simulink model "MPG_MG_freq"  (R2021b)
settings: Solver=VariableStepAuto  StartTime=0.0  StopTime=7  RelTol=1e-3
model workspace (MAT data in the model file):
  Ts : Simulink.Parameter (value not decoded)
  secondary_on : Simulink.Parameter (value not decoded)
values from neighbouring files (symbols this model uses):
  A = zeros(4,4)    [MPC_MG_script_raw_dmpc.m]    (also in MPG_MG_July.m = [0 1 1 1; 1 0 0 0; 1 0 0 0; 1 0 0 0]; MPG_MG_freq_script.m = ones(4) - eye(4); Script.m = [0 1 1 1 ; 1 0 1 1 ; 1 1 0 1 ; 1 1 1 0])
  C_f = 50e-6    (= 5e-05)    [Four_DG_MG_PrimaryOnlyScript.m]    (also in MPC_MG_script.m; MPC_MG_script_raw_dmpc.m; MPC_MG_secondary_script.m; MPG_MG_July.m)
  f_c = 5000    [Four_DG_MG_PrimaryOnlyScript.m]    (also in MPC_MG_script.m = 40000; MPC_MG_script_raw_dmpc.m = 40000; MPC_MG_secondary_script.m = 40000; MPG_MG_July.m = 50000)
  kL = 1e-5    (= 1e-05)    [Four_DG_MG_PrimaryOnlyScript.m]    (also in MPC_MG_script.m = 1e-08; MPC_MG_script_raw_dmpc.m = 1e-08; MPC_MG_secondary_script.m = 1e-07; MPG_MG_July.m = 1e-07)
  L_f = 1.35e-3    (= 0.00135)    [Four_DG_MG_PrimaryOnlyScript.m]    (also in MPC_MG_script.m; MPC_MG_script_raw_dmpc.m; MPC_MG_secondary_script.m; MPG_MG_July.m)
  L_in1 = 0.35e-3    (= 0.00035)    [Four_DG_MG_PrimaryOnlyScript.m]    (also in MPC_MG_script.m; MPC_MG_script_raw_dmpc.m; MPC_MG_secondary_script.m; MPG_MG_July.m)
  L_in2 = 0.35e-3    (= 0.00035)    [Four_DG_MG_PrimaryOnlyScript.m]    (also in MPC_MG_script.m; MPC_MG_script_raw_dmpc.m; MPC_MG_secondary_script.m; MPG_MG_July.m)
  L_in4 = 0.35e-3    (= 0.00035)    [Four_DG_MG_PrimaryOnlyScript.m]    (also in MPC_MG_script.m; MPC_MG_script_raw_dmpc.m; MPC_MG_secondary_script.m; MPG_MG_July.m)
  lambda1 = [30000 50000 90000 50000]'    [MPC_MG_script_raw_dmpc.m]    (also in MPG_MG_July.m = [4 4 4 4]'; MPG_MG_freq_script.m = [3 3 3 3]'; Script.m = [1 1 1 1]')
  lambda2 = [5 6 7 6]'    [MPC_MG_script_raw_dmpc.m]    (also in MPG_MG_July.m = [0.5e-2 0.5e-2 0.5e-2 0.5e-2]'; MPG_MG_freq_script.m = [1.1 1.9 1.5 1.2]'; Script.m = [0.8e-2 0.8e-2 0.8e-2 0.8e-2]')
  lambda3 = [80000 80000 900000 80000]'    [MPC_MG_script_raw_dmpc.m]    (also in MPG_MG_July.m = [1e-3 1e-3 1e-3 1e-3]'; MPG_MG_freq_script.m = [9e-4 1.2e-2 3e-3 3e-3]'; Script.m = [1.5e-3 1.5e-3 1.5e-3 1.5e-3]')
  LD_ref1 = 800e-6    (= 0.0008)    [Four_DG_MG_PrimaryOnlyScript.m]    (also in MPC_MG_script.m = 0.0003; MPC_MG_script_raw_dmpc.m = 0.0003; MPC_MG_secondary_script.m = 0.0001; MPG_MG_July.m = 0.0004)
  lo_co = 0.2    [Four_DG_MG_PrimaryOnlyScript.m]    (also in MPC_MG_script.m = 0.05; MPC_MG_script_raw_dmpc.m; MPC_MG_secondary_script.m = 0.08; MPG_MG_July.m = 0.15)
  m_p1 = 9.4e-5/droopDivide    (= 9.4e-05)    [Four_DG_MG_PrimaryOnlyScript.m]    (also in MPC_MG_script.m; MPC_MG_script_raw_dmpc.m; MPC_MG_secondary_script.m; MPG_MG_July.m)
  m_p2 = 9.4e-5/droopDivide    (= 9.4e-05)    [Four_DG_MG_PrimaryOnlyScript.m]    (also in MPC_MG_script.m; MPC_MG_script_raw_dmpc.m; MPC_MG_secondary_script.m; MPG_MG_July.m)
  m_p3 = 12.5e-5/droopDivide    (= 0.000125)    [Four_DG_MG_PrimaryOnlyScript.m]    (also in MPC_MG_script.m; MPC_MG_script_raw_dmpc.m; MPC_MG_secondary_script.m; MPG_MG_July.m)
  m_p4 = 12.5e-5/droopDivide    (= 0.000125)    [Four_DG_MG_PrimaryOnlyScript.m]    (also in MPC_MG_script.m; MPC_MG_script_raw_dmpc.m; MPC_MG_secondary_script.m; MPG_MG_July.m)
  N = 3    [MPG_MG_July.m]    (also in MPG_MG_freq_script.m; Script.m = 5)
  n_q1 = 1.3e-3/droopDivide2    (= 0.00013)    [Four_DG_MG_PrimaryOnlyScript.m]    (also in MPC_MG_script.m; MPC_MG_script_raw_dmpc.m; MPC_MG_secondary_script.m; MPG_MG_July.m)
  n_q2 = 1.3e-3/droopDivide2    (= 0.00013)    [Four_DG_MG_PrimaryOnlyScript.m]    (also in MPC_MG_script.m; MPC_MG_script_raw_dmpc.m; MPC_MG_secondary_script.m; MPG_MG_July.m)
  n_q4 = 1.5e-3/droopDivide2    (= 0.00015)    [Four_DG_MG_PrimaryOnlyScript.m]    (also in MPC_MG_script.m; MPC_MG_script_raw_dmpc.m; MPC_MG_secondary_script.m; MPG_MG_July.m)
  Pmax = [45e3 45e3 37e3 37e3]'    [MPG_MG_July.m]    (also in MPG_MG_freq_script.m = [4e3 3.5e3 3.5e3 4e3]'; Script.m)
  R_f = 0.1    [Four_DG_MG_PrimaryOnlyScript.m]    (also in MPC_MG_script.m; MPC_MG_script_raw_dmpc.m; MPC_MG_secondary_script.m; MPG_MG_July.m)
  R_in1 = 0.03    [Four_DG_MG_PrimaryOnlyScript.m]    (also in MPC_MG_script.m; MPC_MG_script_raw_dmpc.m; MPC_MG_secondary_script.m; MPG_MG_July.m)
  R_in2 = 0.03    [Four_DG_MG_PrimaryOnlyScript.m]    (also in MPC_MG_script.m; MPC_MG_script_raw_dmpc.m; MPC_MG_secondary_script.m; MPG_MG_July.m)
  R_in4 = 0.03    [Four_DG_MG_PrimaryOnlyScript.m]    (also in MPC_MG_script.m; MPC_MG_script_raw_dmpc.m; MPC_MG_secondary_script.m; MPG_MG_July.m)
  time_thresh = 0.6    [Four_DG_MG_PrimaryOnlyScript.m]    (also in MPC_MG_script_raw_dmpc.m = 1.5; MPC_MG_secondary_script.m = 2; MPG_MG_July.m = 0.5; MPG_MG_freq_script.m = 0.5)
  Ts = 10e-6    (= 1e-05)    [Four_DG_MG_PrimaryOnlyScript.m]    (also in MPC_MG_script.m; MPC_MG_script_raw_dmpc.m; MPC_MG_secondary_script.m; MPG_MG_July.m)
  Tsamp = 0.1    [MPG_MG_July.m]    (also in MPG_MG_freq_script.m; Script.m)
  V_nom = 220*sqrt(2)    [Four_DG_MG_PrimaryOnlyScript.m]    (also in MPC_MG_script.m; MPC_MG_script_raw_dmpc.m; MPC_MG_secondary_script.m; MPG_MG_July.m)
  Vdc = 600    [Four_DG_MG_PrimaryOnlyScript.m]    (also in MPC_MG_script.m; MPC_MG_script_raw_dmpc.m; MPC_MG_secondary_script.m; MPG_MG_July.m)
  w_c_high = 2*pi*50    (= 314.159265359)    [Four_DG_MG_PrimaryOnlyScript.m]    (also in MPC_MG_script.m; MPC_MG_script_raw_dmpc.m; MPC_MG_secondary_script.m; MPG_MG_July.m)
  w_nom = 2*pi*50    (= 314.159265359)    [Four_DG_MG_PrimaryOnlyScript.m]    (also in MPC_MG_script.m; MPC_MG_script_raw_dmpc.m; MPC_MG_secondary_script.m; MPG_MG_July.m)
undefined symbols (not defined in the file or in its folder): i
libraries: spsThreePhaseSeriesRLCBranchLib x18, spsabctodq0Lib x16, spsThreePhaseVIMeasurementLib x15, eeGeneralControl x14, dspswit3 x5, spsDCVoltageSourceLib x5, spsSeriesRLCBranchLib x5, spsTwoLevelConverterLib x5, slpidlib x4, spsThreePhaseSeriesRLCLoadLib x2, spsThreePhaseBreakerLib x2, spsPLL3phLib x2
(part 4 of 4)

== matlab function MPG_MG_freq/Voltage Source Inverter 2/Model Predictive Control  ==
  settings: updateMethod=DISCRETE  sampleTime=Ts
  data: S_opt output; Sopt output size=[1 6]; Vc input; i_filter input; vref input; Vi_opt output; Vdc parameter double size=1; modT parameter size=1; Cfilter parameter size=1; Lfilter parameter size=1
function [S_opt, Sopt, Vi_opt] = MPC(Vc, i_filter,vref,Vdc,modT,Cfilter,Lfilter)

    % In order to call "cont2dis" function
    coder.extrinsic('cont2dis');
    persistent Aq Bq Bdq Vck ifk  Vc_old if_old x_opt g f_window f_window2

    % Initialize variables and get the parameters of the Discrete model based on Ts
    if isempty(x_opt), x_opt = ones(1, 2); end
    if isempty(Vc_old), Vc_old = 0 + 1j*0; end
    if isempty(if_old), if_old = 0 + 1j*0; end
    if isempty(Vck), Vck = ones(1, 4) * (0 + 1j*0); end
    if isempty(ifk), ifk = ones(1, 4) * (0 + 1j*0); end
    if isempty(f_window), f_window = zeros(1,51); end
    if isempty(f_window2), f_window2 = zeros(1,51); end

    if isempty(Aq) && isempty(Bq) && isempty(Bdq)
        Aq = zeros(2);     Bq = zeros(2,1);     Bdq = zeros(2,1);
        % Call "cont2dis" function
        [Aq, Bq, Bdq] = cont2dis(modT,Lfilter,Cfilter); 
    end
    
    % Intialize the cost function
    g_opt = inf;
    
    % To generate the switching states matrix
    states = [1 0 0;
              0 0 0  
              1 1 0
              0 1 0
              0 1 1
              0 0 1
              1 0 1
              1 1 1];
    a = exp(1j*(2*pi/3));
    % Read current measurements at sampling instant k
    ifk(1) = i_filter;
    Vck(1) = Vc;
    % Equation of io(k-1) = if(k-1)-(c/Ts)(vc(k)-vc(k-1)).
    io = ones(1, 3) * (0 + 1j*0);
    io(1) = if_old - (Cfilter/modT)*(Vck(1) - Vc_old); 
    
    % Store the measured current for the next iteration
    if_old = i_filter;
    Vc_old = Vc;
    % FOR loop to find the best switch in the next instant and its corresponding V(i)
    k = ones(1,3);
    s = zeros(3,3);
    sw = zeros(1,3)* (0 + 1j*0);
    Vi = zeros(1,3)* (0 + 1j*0);
    for a1 = 1:8
        k(1) = a1;
        %constraint check
        if (abs(states(k(1),:)-states(x_opt(1),:)) > 1)
            continue
        end
        %state calculation
        s(1,:) = states(k(1),:);
        sw(1) = (2/3)*(s(1,1)+a*s(1,2)+a^2*s(1,3));
        Vi(1) = Vdc*sw(1);

        % Output Voltage Prediction at instant k+1
        ifk(2) = Aq(1,1)*ifk(1) + Aq(1,2)*Vck(1) + Bq(1)*Vi(1) + Bdq(1)*io(1); 
        Vck(2) = Aq(2,1)*ifk(1) + Aq(2,2)*Vck(1) + Bq(2)*Vi(1) + Bdq(2)*io(1); 
        
        for a2 = 1:8
            k(2) = a2;
            %constraint check
            if (abs(states(k(2),:)-states(k(1),:)) > 1)
                continue
            end
            io(2) = io(1) - (Cfilter/modT)*(Vck(2) - Vck(1));
            %state calculation
            s(2,:) = states(k(2),:);
            sw(2) = (2/3)*(s(2,1)+a*s(2,2)+a^2*s(2,3));
            Vi(2) = Vdc*sw(2);
    
            % Output Voltage Prediction at instant k+1
            ifk(3) = Aq(1,1)*ifk(2) + Aq(1,2)*Vck(2) + Bq(1)*Vi(2) + Bdq(1)*io(2); 
            Vck(3) = Aq(2,1)*ifk(2) + Aq(2,2)*Vck(2) + Bq(2)*Vi(2) + Bdq(2)*io(2); 

            g1 = (real(ifk(3))-real(io(3))+Cfilter*2*pi*50*imag(vref))^2 + (imag(ifk(3))-imag(io(3))+Cfilter*2*pi*50*real(vref))^2;
            g = (real(vref)-real(Vck(3)))^2+(imag(vref)-imag(Vck(3)))^2 + 0.1*g1 + 0.1*sum(states(a2)-states(a1),'all')^2;
            if (g<g_opt)
                x_opt = [k(1) k(2)];
                g_opt = g;
            end
           
        end 
    end

     
    
    % Output switching states and its voltage vector. 
    Vi_opt = x_opt(1); 
    S_opt = states(x_opt(1),:);
    d_opt = not(S_opt);
    Sopt = [S_opt,d_opt];     

end

== matlab function MPG_MG_freq/Voltage Source Inverter 1/Model Predictive Control  ==
  settings: updateMethod=DISCRETE  sampleTime=Ts
  data: Sopt output size=[1 6]; Vc input; i_filter input; vref input; Vdc parameter double size=1; modT parameter size=1; Cfilter parameter size=1; Lfilter parameter size=1
function Sopt  = MPC(Vc, i_filter,vref,Vdc,modT,Cfilter,Lfilter)

    % In order to call "cont2dis" function
    coder.extrinsic('cont2dis');
    persistent Aq Bq Bdq Vck ifk  Vc_old if_old x_opt g f_window f_window2

    % Initialize variables and get the parameters of the Discrete model based on Ts
    if isempty(x_opt), x_opt = ones(1, 2); end
    if isempty(Vc_old), Vc_old = 0 + 1j*0; end
    if isempty(if_old), if_old = 0 + 1j*0; end
    if isempty(Vck), Vck = ones(1, 4) * (0 + 1j*0); end
    if isempty(ifk), ifk = ones(1, 4) * (0 + 1j*0); end
    if isempty(f_window), f_window = zeros(1,51); end
    if isempty(f_window2), f_window2 = zeros(1,51); end

    if isempty(Aq) && isempty(Bq) && isempty(Bdq)
        Aq = zeros(2);     Bq = zeros(2,1);     Bdq = zeros(2,1);
        % Call "cont2dis" function
        [Aq, Bq, Bdq] = cont2dis(modT,Lfilter,Cfilter); 
    end
    
    % Intialize the cost function
    g_opt = inf;
    
    % To generate the switching states matrix
    states = [1 0 0;
              0 0 0  
              1 1 0
              0 1 0
              0 1 1
              0 0 1
              1 0 1
              1 1 1];
    a = exp(1j*(2*pi/3));
    % Read current measurements at sampling instant k
    ifk(1) = i_filter;
    Vck(1) = Vc;
    % Equation of io(k-1) = if(k-1)-(c/Ts)(vc(k)-vc(k-1)).
    io = ones(1, 3) * (0 + 1j*0);
    io(1) = if_old - (Cfilter/modT)*(Vck(1) - Vc_old); 
    
    % Store the measured current for the next iteration
    if_old = i_filter;
    Vc_old = Vc;
    % FOR loop to find the best switch in the next instant and its corresponding V(i)
    k = ones(1,3);
    s = zeros(3,3);
    sw = zeros(1,3)* (0 + 1j*0);
    Vi = zeros(1,3)* (0 + 1j*0);
    for a1 = 1:8
        k(1) = a1;
        %constraint check
        if (abs(states(k(1),:)-states(x_opt(1),:)) > 1)
            continue
        end
        %state calculation
        s(1,:) = states(k(1),:);
        sw(1) = (2/3)*(s(1,1)+a*s(1,2)+a^2*s(1,3));
        Vi(1) = Vdc*sw(1);

        % Output Voltage Prediction at instant k+1
        ifk(2) = Aq(1,1)*ifk(1) + Aq(1,2)*Vck(1) + Bq(1)*Vi(1) + Bdq(1)*io(1); 
        Vck(2) = Aq(2,1)*ifk(1) + Aq(2,2)*Vck(1) + Bq(2)*Vi(1) + Bdq(2)*io(1); 
        
        for a2 = 1:8
            k(2) = a2;
            %constraint check
            if (abs(states(k(2),:)-states(k(1),:)) > 1)
                continue
            end
            io(2) = io(1) - (Cfilter/modT)*(Vck(2) - Vck(1));
            %state calculation
            s(2,:) = states(k(2),:);
            sw(2) = (2/3)*(s(2,1)+a*s(2,2)+a^2*s(2,3));
            Vi(2) = Vdc*sw(2);
    
            % Output Voltage Prediction at instant k+1
            ifk(3) = Aq(1,1)*ifk(2) + Aq(1,2)*Vck(2) + Bq(1)*Vi(2) + Bdq(1)*io(2); 
            Vck(3) = Aq(2,1)*ifk(2) + Aq(2,2)*Vck(2) + Bq(2)*Vi(2) + Bdq(2)*io(2); 

            g1 = (real(ifk(3))-real(io(3))+Cfilter*2*pi*50*imag(vref))^2 + (imag(ifk(3))-imag(io(3))+Cfilter*2*pi*50*real(vref))^2;
            g = (real(vref)-real(Vck(3)))^2+(imag(vref)-imag(Vck(3)))^2 + 0.1*g1;
            if (g<g_opt)
                x_opt = [k(1) k(2)];
                g_opt = g;
            end
           
        end 
    end

     
    
    % Output switching states and its voltage vector. 
    Vi_opt = x_opt(1); 
    S_opt = states(x_opt(1),:);
    d_opt = not(S_opt);
    Sopt = [S_opt,d_opt];     

end

== matlab function MPG_MG_freq/Voltage Source Inverter 3/Model Predictive Control  ==
  settings: updateMethod=DISCRETE  sampleTime=Ts
  data: S_opt output; Sopt output size=[1 6]; Vc input; i_filter input; vref input; Vi_opt output; Vdc parameter double size=1; modT parameter size=1; Cfilter parameter size=1; Lfilter parameter size=1
function [S_opt, Sopt, Vi_opt] = MPC(Vc, i_filter,vref,Vdc,modT,Cfilter,Lfilter)

    % In order to call "cont2dis" function
    coder.extrinsic('cont2dis');
    persistent Aq Bq Bdq Vck ifk  Vc_old if_old x_opt g f_window f_window2

    % Initialize variables and get the parameters of the Discrete model based on Ts
    if isempty(x_opt), x_opt = ones(1, 2); end
    if isempty(Vc_old), Vc_old = 0 + 1j*0; end
    if isempty(if_old), if_old = 0 + 1j*0; end
    if isempty(Vck), Vck = ones(1, 4) * (0 + 1j*0); end
    if isempty(ifk), ifk = ones(1, 4) * (0 + 1j*0); end
    if isempty(f_window), f_window = zeros(1,51); end
    if isempty(f_window2), f_window2 = zeros(1,51); end

    if isempty(Aq) && isempty(Bq) && isempty(Bdq)
        Aq = zeros(2);     Bq = zeros(2,1);     Bdq = zeros(2,1);
        % Call "cont2dis" function
        [Aq, Bq, Bdq] = cont2dis(modT,Lfilter,Cfilter); 
    end
    
    % Intialize the cost function
    g_opt = inf;
    
    % To generate the switching states matrix
    states = [1 0 0;
              0 0 0  
              1 1 0
              0 1 0
              0 1 1
              0 0 1
              1 0 1
              1 1 1];
    a = exp(1j*(2*pi/3));
    % Read current measurements at sampling instant k
    ifk(1) = i_filter;
    Vck(1) = Vc;
    % Equation of io(k-1) = if(k-1)-(c/Ts)(vc(k)-vc(k-1)).
    io = ones(1, 3) * (0 + 1j*0);
    io(1) = if_old - (Cfilter/modT)*(Vck(1) - Vc_old); 
    
    % Store the measured current for the next iteration
    if_old = i_filter;
    Vc_old = Vc;
    % FOR loop to find the best switch in the next instant and its corresponding V(i)
    k = ones(1,3);
    s = zeros(3,3);
    sw = zeros(1,3)* (0 + 1j*0);
    Vi = zeros(1,3)* (0 + 1j*0);
    for a1 = 1:8
        k(1) = a1;
        %constraint check
        if (abs(states(k(1),:)-states(x_opt(1),:)) > 1)
            continue
        end
        %state calculation
        s(1,:) = states(k(1),:);
        sw(1) = (2/3)*(s(1,1)+a*s(1,2)+a^2*s(1,3));
        Vi(1) = Vdc*sw(1);

        % Output Voltage Prediction at instant k+1
        ifk(2) = Aq(1,1)*ifk(1) + Aq(1,2)*Vck(1) + Bq(1)*Vi(1) + Bdq(1)*io(1); 
        Vck(2) = Aq(2,1)*ifk(1) + Aq(2,2)*Vck(1) + Bq(2)*Vi(1) + Bdq(2)*io(1); 
        
        for a2 = 1:8
            k(2) = a2;
            %constraint check
            if (abs(states(k(2),:)-states(k(1),:)) > 1)
                continue
            end
            io(2) = io(1) - (Cfilter/modT)*(Vck(2) - Vck(1));
            %state calculation
            s(2,:) = states(k(2),:);
            sw(2) = (2/3)*(s(2,1)+a*s(2,2)+a^2*s(2,3));
            Vi(2) = Vdc*sw(2);
    
            % Output Voltage Prediction at instant k+1
            ifk(3) = Aq(1,1)*ifk(2) + Aq(1,2)*Vck(2) + Bq(1)*Vi(2) + Bdq(1)*io(2); 
            Vck(3) = Aq(2,1)*ifk(2) + Aq(2,2)*Vck(2) + Bq(2)*Vi(2) + Bdq(2)*io(2); 

            g1 = (real(ifk(3))-real(io(3))+Cfilter*2*pi*50*imag(vref))^2 + (imag(ifk(3))-imag(io(3))+Cfilter*2*pi*50*real(vref))^2;
            g = (real(vref)-real(Vck(3)))^2+(imag(vref)-imag(Vck(3)))^2 + 0.1*g1 + 0.1*sum(states(a2)-states(a1),'all')^2;
            if (g<g_opt)
                x_opt = [k(1) k(2)];
                g_opt = g;
            end
           
        end 
    end

     
    
    % Output switching states and its voltage vector. 
    Vi_opt = x_opt(1); 
    S_opt = states(x_opt(1),:);
    d_opt = not(S_opt);
    Sopt = [S_opt,d_opt];     

end

== matlab function MPG_MG_freq/MPC-based Secondary Controller/Subsystem1/Model Predictive Control 1 ==
  settings: updateMethod=DISCRETE  sampleTime=Ts
  data: flag output; X input; a input; x_out output; L_f input; Mpw input; Tsec input; omega input; omega_s input; V input; V_s input; theta input; P input; w_nom input; lambda1 input; lambda2 input; lambda3 input; Pmax input; aij input; N parameter
function [flag, x_out] = dmpc(X, a, L_f, Mpw, Tsec, omega, omega_s, V, V_s, theta, P, w_nom, lambda1, lambda2, lambda3, Pmax, aij, N)
    %step 5: update matrices
   
    Ai = zeros(2*N,5*N);

    Ai(1:N,(4*N+1):5*N) = -eye(N);
    Ai((1*N+1):2*N,(4*N+1):5*N) = eye(N);

    Bi = zeros((2*N),1);

    Bi((1+N):(2*N),1) = Pmax(a)*ones(N,1);

    tz = toeplitz([1 -1 zeros(1,N-2)], [1 zeros(1,N-1)]);

    Aeq = zeros(4*N,5*N);

    Aeq((N+1):2*N, (N+1):(2*N)) = -eye(N);
    Aeq((N+1):2*N, (2*N+1):3*N) = tz;
    Aeq((N+1):2*N, (4*N+1):5*N) =  -Mpw*tz;

    Aeq((2*N+1):(3*N), (2*N+1):(3*N)) = -Tsec*eye(N); 
    Aeq((2*N+1):(3*N), (3*N+1):4*N) = tz;

    Aeq((3*N+1):(4*N), (3*N+1):(4*N)) = -V(a)*V_s(a)*cos(theta(a))/(L_f*w_nom)*eye(N);
    Aeq((3*N+1):(4*N), (4*N+1):5*N) = eye(N);

    I9 = eye(N);
    I9(N,N) = 0;

    Aeq(1:N, 1:N) = eye(N);
    Aeq(1:N, (2*N+1):(3*N)) = -1/(1+sum(aij(a,:)))*I9;
   
    Beq = zeros(4*N,1);

    Beq(1:N,1) = (aij(a,:)*X(:,(2*N+1):3*N)./(1+sum(aij(a,:))))';

    Beq(N+1,1) = omega(a)-Mpw*P(a);

    Beq((2*N+1),1) = theta(a)-Tsec*omega_s(a);
    Beq((2*N+2):(3*N),1) = -Tsec*omega_s(a)*ones((N-1),1);

    Beq((3*N+1):(4*N),1) = (P(a)-theta(a)*V(a)*V_s(a)*cos(theta(a))/(L_f*w_nom))*ones(N,1);
    
    H = zeros(5*N);
    H(1:N,1:N) = 2*lambda1(a)*eye(N);
    H((N+1):(2*N),(N+1):(2*N)) = 2*lambda2(a)*eye(N);
    H((4*N+1):5*N,(4*N+1):5*N) = 2*lambda3(a)*sum(aij(a,:))/(Pmax(a)^2)*eye(N);

    S_pred = ones(4,N);
    for k = 1:N
        S_pred(:,k) = Pmax; 
    end

    F = zeros(5*N,1);
    F(1:N,1) = -2*lambda1(a)*w_nom*ones(N,1);

    F((4*N+1):5*N,1) = -2*lambda3(a)*(aij(a,:)*(X(:,(4*N+1):5*N)./(S_pred))/Pmax(a))';
    %P_pred 4x10 matrix
    options = optimoptions('quadprog', 'Algorithm','active-set');
    %required initial point x0
    %   OPTIMIZE
    x0 = zeros(5*N,1);
    x0(1,1) = w_nom;
    x0((N+1),1) = 0;
    x0((2*N+1),1) = w_nom;
    x0((3*N+1),1) = 0.963;
    x0((4*N+1),1) = 0;

    [x,~,exitflag] = quadprog(H, F, Ai, Bi, Aeq, Beq, [], [], x0, options);
    x_out = x;

    if exitflag < 1
       x((N+1),1) = 0;
    else
        x_out = x;
    end
    flag = exitflag;
end

== matlab function MPG_MG_freq/MPC-based Secondary Controller/Subsystem6/Model Predictive Control 1 ==
  settings: updateMethod=DISCRETE  sampleTime=Ts
  data: flag output; X input; a input; x_out output; L_f input; Mpw input; Tsec input; omega input; omega_s input; V input; V_s input; theta input; P input; w_nom input; lambda1 input; lambda2 input; lambda3 input; Pmax input; aij input; N parameter
function [flag, x_out] = dmpc(X, a, L_f, Mpw, Tsec, omega, omega_s, V, V_s, theta, P, w_nom, lambda1, lambda2, lambda3, Pmax, aij, N)
    %step 5: update matrices
   
    Ai = zeros(2*N,5*N);

    Ai(1:N,(4*N+1):5*N) = -eye(N);
    Ai((1*N+1):2*N,(4*N+1):5*N) = eye(N);

    Bi = zeros((2*N),1);

    Bi((1+N):(2*N),1) = Pmax(a)*ones(N,1);

    tz = toeplitz([1 -1 zeros(1,N-2)], [1 zeros(1,N-1)]);

    Aeq = zeros(4*N,5*N);

    Aeq((N+1):2*N, (N+1):(2*N)) = -eye(N);
    Aeq((N+1):2*N, (2*N+1):3*N) = tz;
    Aeq((N+1):2*N, (4*N+1):5*N) =  -Mpw*tz;

    Aeq((2*N+1):(3*N), (2*N+1):(3*N)) = -Tsec*eye(N); 
    Aeq((2*N+1):(3*N), (3*N+1):4*N) = tz;

    Aeq((3*N+1):(4*N), (3*N+1):(4*N)) = -V(a)*V_s(a)*cos(theta(a))/(L_f*w_nom)*eye(N);
    Aeq((3*N+1):(4*N), (4*N+1):5*N) = eye(N);

    I9 = eye(N);
    I9(N,N) = 0;

    Aeq(1:N, 1:N) = eye(N);
    Aeq(1:N, (2*N+1):(3*N)) = -1/(1+sum(aij(a,:)))*I9;
   
    Beq = zeros(4*N,1);

    Beq(1:N,1) = (aij(a,:)*X(:,(2*N+1):3*N)./(1+sum(aij(a,:))))';

    Beq(N+1,1) = omega(a)-Mpw*P(a);

    Beq((2*N+1),1) = theta(a)-Tsec*omega_s(a);
    Beq((2*N+2):(3*N),1) = -Tsec*omega_s(a)*ones((N-1),1);

    Beq((3*N+1):(4*N),1) = (P(a)-theta(a)*V(a)*V_s(a)*cos(theta(a))/(L_f*w_nom))*ones(N,1);
    
    H = zeros(5*N);
    H(1:N,1:N) = 2*lambda1(a)*eye(N);
    H((N+1):(2*N),(N+1):(2*N)) = 2*lambda2(a)*eye(N);
    H((4*N+1):5*N,(4*N+1):5*N) = 2*lambda3(a)*sum(aij(a,:))/(Pmax(a)^2)*eye(N);

    S_pred = ones(4,N);
    for k = 1:N
        S_pred(:,k) = Pmax; 
    end

    F = zeros(5*N,1);
    F(1:N,1) = -2*lambda1(a)*w_nom*ones(N,1);

    F((4*N+1):5*N,1) = -2*lambda3(a)*(aij(a,:)*(X(:,(4*N+1):5*N)./(S_pred))/Pmax(a))';
    %P_pred 4x10 matrix
    options = optimoptions('quadprog', 'Algorithm','active-set');
    %required initial point x0
    %   OPTIMIZE
    x0 = zeros(5*N,1);
    x0(1,1) = w_nom;
    x0((N+1),1) = 0;
    x0((2*N+1),1) = w_nom;
    x0((3*N+1),1) = 0.963;
    x0((4*N+1),1) = 0;

    [x,~,exitflag] = quadprog(H, F, Ai, Bi, Aeq, Beq, [], [], x0, options);
    x_out = x;

    if exitflag < 1
       x((N+1),1) = 0;
    else
        x_out = x;
    end
    flag = exitflag;
end

== matlab function MPG_MG_freq/Voltage Source Inverter 4/Model Predictive Control  ==
  settings: updateMethod=DISCRETE  sampleTime=Ts
  data: S_opt output; Sopt output size=[1 6]; Vc input; i_filter input; vref input; Vi_opt output; Vdc parameter double size=1; modT parameter size=1; Cfilter parameter size=1; Lfilter parameter size=1
function [S_opt, Sopt, Vi_opt] = MPC(Vc, i_filter,vref,Vdc,modT,Cfilter,Lfilter)

    % In order to call "cont2dis" function
    coder.extrinsic('cont2dis');
    persistent Aq Bq Bdq Vck ifk  Vc_old if_old x_opt g f_window f_window2

    % Initialize variables and get the parameters of the Discrete model based on Ts
    if isempty(x_opt), x_opt = ones(1, 2); end
    if isempty(Vc_old), Vc_old = 0 + 1j*0; end
    if isempty(if_old), if_old = 0 + 1j*0; end
    if isempty(Vck), Vck = ones(1, 4) * (0 + 1j*0); end
    if isempty(ifk), ifk = ones(1, 4) * (0 + 1j*0); end
    if isempty(f_window), f_window = zeros(1,51); end
    if isempty(f_window2), f_window2 = zeros(1,51); end

    if isempty(Aq) && isempty(Bq) && isempty(Bdq)
        Aq = zeros(2);     Bq = zeros(2,1);     Bdq = zeros(2,1);
        % Call "cont2dis" function
        [Aq, Bq, Bdq] = cont2dis(modT,Lfilter,Cfilter); 
    end
    
    % Intialize the cost function
    g_opt = inf;
    
    % To generate the switching states matrix
    states = [1 0 0;
              0 0 0  
              1 1 0
              0 1 0
              0 1 1
              0 0 1
              1 0 1
              1 1 1];
    a = exp(1j*(2*pi/3));
    % Read current measurements at sampling instant k
    ifk(1) = i_filter;
    Vck(1) = Vc;
    % Equation of io(k-1) = if(k-1)-(c/Ts)(vc(k)-vc(k-1)).
    io = ones(1, 3) * (0 + 1j*0);
    io(1) = if_old - (Cfilter/modT)*(Vck(1) - Vc_old); 
    
    % Store the measured current for the next iteration
    if_old = i_filter;
    Vc_old = Vc;
    % FOR loop to find the best switch in the next instant and its corresponding V(i)
    k = ones(1,3);
    s = zeros(3,3);
    sw = zeros(1,3)* (0 + 1j*0);
    Vi = zeros(1,3)* (0 + 1j*0);
    for a1 = 1:8
        k(1) = a1;
        %constraint check
        if (abs(states(k(1),:)-states(x_opt(1),:)) > 1)
            continue
        end
        %state calculation
        s(1,:) = states(k(1),:);
        sw(1) = (2/3)*(s(1,1)+a*s(1,2)+a^2*s(1,3));
        Vi(1) = Vdc*sw(1);

        % Output Voltage Prediction at instant k+1
        ifk(2) = Aq(1,1)*ifk(1) + Aq(1,2)*Vck(1) + Bq(1)*Vi(1) + Bdq(1)*io(1); 
        Vck(2) = Aq(2,1)*ifk(1) + Aq(2,2)*Vck(1) + Bq(2)*Vi(1) + Bdq(2)*io(1); 
        
        for a2 = 1:8
            k(2) = a2;
            %constraint check
            if (abs(states(k(2),:)-states(k(1),:)) > 1)
                continue
            end
            io(2) = io(1) - (Cfilter/modT)*(Vck(2) - Vck(1));
            %state calculation
            s(2,:) = states(k(2),:);
            sw(2) = (2/3)*(s(2,1)+a*s(2,2)+a^2*s(2,3));
            Vi(2) = Vdc*sw(2);
    
            % Output Voltage Prediction at instant k+1
            ifk(3) = Aq(1,1)*ifk(2) + Aq(1,2)*Vck(2) + Bq(1)*Vi(2) + Bdq(1)*io(2); 
            Vck(3) = Aq(2,1)*ifk(2) + Aq(2,2)*Vck(2) + Bq(2)*Vi(2) + Bdq(2)*io(2); 

            g1 = (real(ifk(3))-real(io(3))+Cfilter*2*pi*50*imag(vref))^2 + (imag(ifk(3))-imag(io(3))+Cfilter*2*pi*50*real(vref))^2;
            g = (real(vref)-real(Vck(3)))^2+(imag(vref)-imag(Vck(3)))^2 + 0.1*g1 + 0.1*sum(states(a2)-states(a1),'all')^2;
            if (g<g_opt)
                x_opt = [k(1) k(2)];
                g_opt = g;
            end
           
        end 
    end

     
    
    % Output switching states and its voltage vector. 
    Vi_opt = x_opt(1); 
    S_opt = states(x_opt(1),:);
    d_opt = not(S_opt);
    Sopt = [S_opt,d_opt];     

end

== matlab function MPG_MG_freq/Voltage Source Inverter 5/Model Predictive Control  ==
  settings: updateMethod=DISCRETE  sampleTime=Ts
  data: S_opt output; Sopt output size=[1 6]; Vc input; i_filter input; vref input; Vi_opt output; Vdc parameter double size=1; modT parameter size=1; Cfilter parameter size=1; Lfilter parameter size=1
function [S_opt, Sopt, Vi_opt] = MPC(Vc, i_filter,vref,Vdc,modT,Cfilter,Lfilter)

    % In order to call "cont2dis" function
    coder.extrinsic('cont2dis');
    persistent Aq Bq Bdq Vck ifk  Vc_old if_old x_opt g f_window f_window2

    % Initialize variables and get the parameters of the Discrete model based on Ts
    if isempty(x_opt), x_opt = ones(1, 2); end
    if isempty(Vc_old), Vc_old = 0 + 1j*0; end
    if isempty(if_old), if_old = 0 + 1j*0; end
    if isempty(Vck), Vck = ones(1, 4) * (0 + 1j*0); end
    if isempty(ifk), ifk = ones(1, 4) * (0 + 1j*0); end
    if isempty(f_window), f_window = zeros(1,51); end
    if isempty(f_window2), f_window2 = zeros(1,51); end

    if isempty(Aq) && isempty(Bq) && isempty(Bdq)
        Aq = zeros(2);     Bq = zeros(2,1);     Bdq = zeros(2,1);
        % Call "cont2dis" function
        [Aq, Bq, Bdq] = cont2dis(modT,Lfilter,Cfilter); 
    end
    
    % Intialize the cost function
    g_opt = inf;
    
    % To generate the switching states matrix
    states = [1 0 0;
              0 0 0  
              1 1 0
              0 1 0
              0 1 1
              0 0 1
              1 0 1
              1 1 1];
    a = exp(1j*(2*pi/3));
    % Read current measurements at sampling instant k
    ifk(1) = i_filter;
    Vck(1) = Vc;
    % Equation of io(k-1) = if(k-1)-(c/Ts)(vc(k)-vc(k-1)).
    io = ones(1, 3) * (0 + 1j*0);
    io(1) = if_old - (Cfilter/modT)*(Vck(1) - Vc_old); 
    
    % Store the measured current for the next iteration
    if_old = i_filter;
    Vc_old = Vc;
    % FOR loop to find the best switch in the next instant and its corresponding V(i)
    k = ones(1,3);
    s = zeros(3,3);
    sw = zeros(1,3)* (0 + 1j*0);
    Vi = zeros(1,3)* (0 + 1j*0);
    for a1 = 1:8
        k(1) = a1;
        %constraint check
        if (abs(states(k(1),:)-states(x_opt(1),:)) > 1)
            continue
        end
        %state calculation
        s(1,:) = states(k(1),:);
        sw(1) = (2/3)*(s(1,1)+a*s(1,2)+a^2*s(1,3));
        Vi(1) = Vdc*sw(1);

        % Output Voltage Prediction at instant k+1
        ifk(2) = Aq(1,1)*ifk(1) + Aq(1,2)*Vck(1) + Bq(1)*Vi(1) + Bdq(1)*io(1); 
        Vck(2) = Aq(2,1)*ifk(1) + Aq(2,2)*Vck(1) + Bq(2)*Vi(1) + Bdq(2)*io(1); 
        
        for a2 = 1:8
            k(2) = a2;
            %constraint check
            if (abs(states(k(2),:)-states(k(1),:)) > 1)
                continue
            end
            io(2) = io(1) - (Cfilter/modT)*(Vck(2) - Vck(1));
            %state calculation
            s(2,:) = states(k(2),:);
            sw(2) = (2/3)*(s(2,1)+a*s(2,2)+a^2*s(2,3));
            Vi(2) = Vdc*sw(2);
    
            % Output Voltage Prediction at instant k+1
            ifk(3) = Aq(1,1)*ifk(2) + Aq(1,2)*Vck(2) + Bq(1)*Vi(2) + Bdq(1)*io(2); 
            Vck(3) = Aq(2,1)*ifk(2) + Aq(2,2)*Vck(2) + Bq(2)*Vi(2) + Bdq(2)*io(2); 

            g1 = (real(ifk(3))-real(io(3))+Cfilter*2*pi*50*imag(vref))^2 + (imag(ifk(3))-imag(io(3))+Cfilter*2*pi*50*real(vref))^2;
            g = (real(vref)-real(Vck(3)))^2+(imag(vref)-imag(Vck(3)))^2 + 0.1*g1 + 0.1*sum(states(a2)-states(a1),'all')^2;
            if (g<g_opt)
                x_opt = [k(1) k(2)];
                g_opt = g;
            end
           
        end 
    end

     
    
    % Output switching states and its voltage vector. 
    Vi_opt = x_opt(1); 
    S_opt = states(x_opt(1),:);
    d_opt = not(S_opt);
    Sopt = [S_opt,d_opt];     

end

== matlab function MPG_MG_freq/MPC-based Secondary Controller/Subsystem5/Model Predictive Control 1 ==
  settings: updateMethod=DISCRETE  sampleTime=Ts
  data: flag output; X input; a input; x_out output; L_f input; Mpw input; Tsec input; omega input; omega_s input; V input; V_s input; theta input; P input; w_nom input; lambda1 input; lambda2 input; lambda3 input; Pmax input; aij input; N parameter
function [flag, x_out] = dmpc(X, a, L_f, Mpw, Tsec, omega, omega_s, V, V_s, theta, P, w_nom, lambda1, lambda2, lambda3, Pmax, aij, N)
    %step 5: update matrices
   
    Ai = zeros(2*N,5*N);

    Ai(1:N,(4*N+1):5*N) = -eye(N);
    Ai((1*N+1):2*N,(4*N+1):5*N) = eye(N);

    Bi = zeros((2*N),1);

    Bi((1+N):(2*N),1) = Pmax(a)*ones(N,1);

    tz = toeplitz([1 -1 zeros(1,N-2)], [1 zeros(1,N-1)]);

    Aeq = zeros(4*N,5*N);

    Aeq((N+1):2*N, (N+1):(2*N)) = -eye(N);
    Aeq((N+1):2*N, (2*N+1):3*N) = tz;
    Aeq((N+1):2*N, (4*N+1):5*N) =  -Mpw*tz;

    Aeq((2*N+1):(3*N), (2*N+1):(3*N)) = -Tsec*eye(N); 
    Aeq((2*N+1):(3*N), (3*N+1):4*N) = tz;

    Aeq((3*N+1):(4*N), (3*N+1):(4*N)) = -V(a)*V_s(a)*cos(theta(a))/(L_f*w_nom)*eye(N);
    Aeq((3*N+1):(4*N), (4*N+1):5*N) = eye(N);

    I9 = eye(N);
    I9(N,N) = 0;

    Aeq(1:N, 1:N) = eye(N);
    Aeq(1:N, (2*N+1):(3*N)) = -1/(1+sum(aij(a,:)))*I9;
   
    Beq = zeros(4*N,1);

    Beq(1:N,1) = (aij(a,:)*X(:,(2*N+1):3*N)./(1+sum(aij(a,:))))';

    Beq(N+1,1) = omega(a)-Mpw*P(a);

    Beq((2*N+1),1) = theta(a)-Tsec*omega_s(a);
    Beq((2*N+2):(3*N),1) = -Tsec*omega_s(a)*ones((N-1),1);

    Beq((3*N+1):(4*N),1) = (P(a)-theta(a)*V(a)*V_s(a)*cos(theta(a))/(L_f*w_nom))*ones(N,1);
    
    H = zeros(5*N);
    H(1:N,1:N) = 2*lambda1(a)*eye(N);
    H((N+1):(2*N),(N+1):(2*N)) = 2*lambda2(a)*eye(N);
    H((4*N+1):5*N,(4*N+1):5*N) = 2*lambda3(a)*sum(aij(a,:))/(Pmax(a)^2)*eye(N);

    S_pred = ones(4,N);
    for k = 1:N
        S_pred(:,k) = Pmax; 
    end

    F = zeros(5*N,1);
    F(1:N,1) = -2*lambda1(a)*w_nom*ones(N,1);

    F((4*N+1):5*N,1) = -2*lambda3(a)*(aij(a,:)*(X(:,(4*N+1):5*N)./(S_pred))/Pmax(a))';
    %P_pred 4x10 matrix
    options = optimoptions('quadprog', 'Algorithm','active-set');
    %required initial point x0
    %   OPTIMIZE
    x0 = zeros(5*N,1);
    x0(1,1) = w_nom;
    x0((N+1),1) = 0;
    x0((2*N+1),1) = w_nom;
    x0((3*N+1),1) = 0.963;
    x0((4*N+1),1) = 0;

    [x,~,exitflag] = quadprog(H, F, Ai, Bi, Aeq, Beq, [], [], x0, options);
    x_out = x;

    if exitflag < 1
       x((N+1),1) = 0;
    else
        x_out = x;
    end
    flag = exitflag;
end

== matlab function MPG_MG_freq/MPC-based Secondary Controller/Subsystem7/Model Predictive Control 1 ==
  settings: updateMethod=DISCRETE  sampleTime=Ts
  data: flag output; X input; a input; x_out output; L_f input; Mpw input; Tsec input; omega input; omega_s input; V input; V_s input; theta input; P input; w_nom input; lambda1 input; lambda2 input; lambda3 input; Pmax input; aij input; N parameter
function [flag, x_out] = dmpc(X, a, L_f, Mpw, Tsec, omega, omega_s, V, V_s, theta, P, w_nom, lambda1, lambda2, lambda3, Pmax, aij, N)
    %step 5: update matrices
   
    Ai = zeros(2*N,5*N);

    Ai(1:N,(4*N+1):5*N) = -eye(N);
    Ai((1*N+1):2*N,(4*N+1):5*N) = eye(N);

    Bi = zeros((2*N),1);

    Bi((1+N):(2*N),1) = Pmax(a)*ones(N,1);

    tz = toeplitz([1 -1 zeros(1,N-2)], [1 zeros(1,N-1)]);

    Aeq = zeros(4*N,5*N);

    Aeq((N+1):2*N, (N+1):(2*N)) = -eye(N);
    Aeq((N+1):2*N, (2*N+1):3*N) = tz;
    Aeq((N+1):2*N, (4*N+1):5*N) =  -Mpw*tz;

    Aeq((2*N+1):(3*N), (2*N+1):(3*N)) = -Tsec*eye(N); 
    Aeq((2*N+1):(3*N), (3*N+1):4*N) = tz;

    Aeq((3*N+1):(4*N), (3*N+1):(4*N)) = -V(a)*V_s(a)*cos(theta(a))/(L_f*w_nom)*eye(N);
    Aeq((3*N+1):(4*N), (4*N+1):5*N) = eye(N);

    I9 = eye(N);
    I9(N,N) = 0;

    Aeq(1:N, 1:N) = eye(N);
    Aeq(1:N, (2*N+1):(3*N)) = -1/(1+sum(aij(a,:)))*I9;
   
    Beq = zeros(4*N,1);

    Beq(1:N,1) = (aij(a,:)*X(:,(2*N+1):3*N)./(1+sum(aij(a,:))))';

    Beq(N+1,1) = omega(a)-Mpw*P(a);

    Beq((2*N+1),1) = theta(a)-Tsec*omega_s(a);
    Beq((2*N+2):(3*N),1) = -Tsec*omega_s(a)*ones((N-1),1);

    Beq((3*N+1):(4*N),1) = (P(a)-theta(a)*V(a)*V_s(a)*cos(theta(a))/(L_f*w_nom))*ones(N,1);
    
    H = zeros(5*N);
    H(1:N,1:N) = 2*lambda1(a)*eye(N);
    H((N+1):(2*N),(N+1):(2*N)) = 2*lambda2(a)*eye(N);
    H((4*N+1):5*N,(4*N+1):5*N) = 2*lambda3(a)*sum(aij(a,:))/(Pmax(a)^2)*eye(N);

    S_pred = ones(4,N);
    for k = 1:N
        S_pred(:,k) = Pmax; 
    end

    F = zeros(5*N,1);
    F(1:N,1) = -2*lambda1(a)*w_nom*ones(N,1);

    F((4*N+1):5*N,1) = -2*lambda3(a)*(aij(a,:)*(X(:,(4*N+1):5*N)./(S_pred))/Pmax(a))';
    %P_pred 4x10 matrix
    options = optimoptions('quadprog', 'Algorithm','active-set');
    %required initial point x0
    %   OPTIMIZE
    x0 = zeros(5*N,1);
    x0(1,1) = w_nom;
    x0((N+1),1) = 0;
    x0((2*N+1),1) = w_nom;
    x0((3*N+1),1) = 0.963;
    x0((4*N+1),1) = 0;

    [x,~,exitflag] = quadprog(H, F, Ai, Bi, Aeq, Beq, [], [], x0, options);
    x_out = x;

    if exitflag < 1
       x((N+1),1) = 0;
    else
        x_out = x;
    end
    flag = exitflag;
end
